simulink model "Calculator_subSys"  (R2016b)
settings: Solver=FixedStepDiscrete  StartTime=0.0  StopTime=10.0  RelTol=1e-3
settings Model: Creator=Rasha  LastModifiedBy=Rasha
settings OptimizationCC: DefaultParameterBehavior=Inlined
settings DebuggingCC: ParameterTunabilityLossMsg=error
settings RTWCC: SystemTargetFile=ert.tlc  GenCodeOnly=on  TemplateMakefile=ert_default_tmf  Description=Embedded Coder  GenerateReport=on  IncludeHyperlinkInReport=on  LaunchReport=on  GenerateTraceInfo=on  GenerateTraceReport=on  GenerateTraceReportSl=on  GenerateTraceReportSf=on  GenerateTraceReportEml=on
settings CodeAppCC: ForceParamTrailComments=on  IgnoreCustomStorageClasses=off  OperatorAnnotations=on  SimulinkDataObjDesc=on  SFDataObjDesc=on  MATLABFcnDesc=on  InsertBlockDesc=on  MATLABSourceComments=on
settings ERTTargetCC: TargetLangStandard=C99 (ISO)  GenerateSampleERTMain=on  InlinedParameterPlacement=NonHierarchical  ERTCustomFileTemplate=example_file_process.tlc

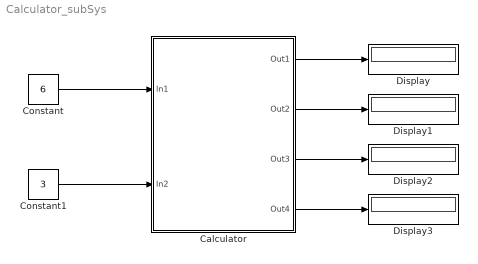
== system Calculator_subSys ==
  Calculator : Subsystem
  Constant : Constant  Value=6
  Constant1 : Constant  Value=3
  Display{,1..3} (4 alike) : Display
  wires:
  Constant/1 -> Calculator/1(In1)
  Constant1/1 -> Calculator/2(In2)
  Calculator/1(Out1) -> Display/1
  Calculator/2(Out2) -> Display1/1
  Calculator/3(Out3) -> Display2/1
  Calculator/4(Out4) -> Display3/1

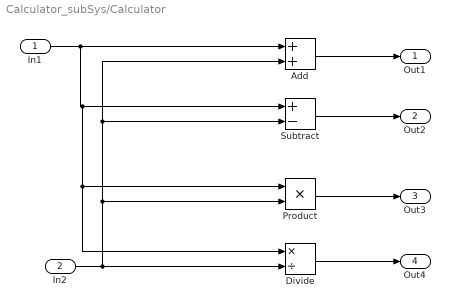
== system Calculator_subSys/Calculator ==
  In1 : Inport
  In2 : Inport  Port=2
  Add : Sum
  Divide : Product  Inputs=*/
  Product : Product
  Subtract : Sum  Inputs=+-
  Out1 : Outport
  Out2 : Outport  Port=2
  Out3 : Outport  Port=3
  Out4 : Outport  Port=4
  wires:
  Divide/1 -> Out4/1
  In2/1 -> Add/2, Subtract/2, Product/2, Divide/2
  In1/1 -> Add/1, Product/1, Divide/1, Subtract/1
  Product/1 -> Out3/1
  Subtract/1 -> Out2/1
  Add/1 -> Out1/1
